simulink model "Simulacao"  (Simulink 8.2)
settings: Solver=ode4  SolverMode=SingleTasking  StartTime=0.0  StopTime=20  FixedStep=0.01  RelTol=1e-3
InitFcn:
  | Main
values from neighbouring files (symbols this model uses):
  T = 1    [Main.m]
  xk0 = [3; 5]    [Main.m]
undefined symbols (not defined in the file or in its folder): A1, B1, C, D
undefined symbols (not defined in the file): A, B, Umax
settings Model: Creator=Kawakami  LastModifiedBy=Eduardo
settings DataIOCC: LimitDataPoints=off  SaveOutput=off  SaveTime=off  TimeSaveName=t  SignalLoggingName=sigsOut
settings OptimizationCC: BooleanDataType=off
settings DebuggingCC: SaveWithParameterizedLinksMsg=none  SignalResolutionControl=TryResolveAllWithWarning  SolverPrmCheckMsg=none  MultiTaskDSMMsg=warning  MultiTaskCondExecSysMsg=none
settings HardwareCC: TargetUnknown=on
settings RTWCC: IncludeERTFirstTime=on

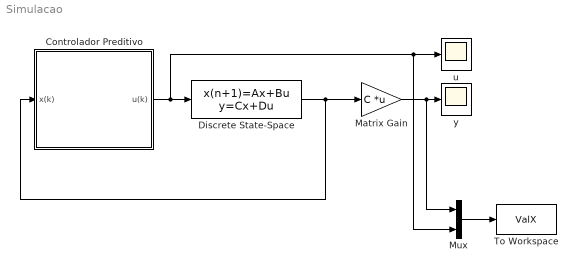
== system Simulacao ==
  "Controlador Preditivo  " : Subsystem  mask{A=A, B=B, Umax=Umax, T=T}
      mask prompts: A "Matriz Agregada A"; B "Matriz Agregada B"; Umax "Input Max"; T "T (passo da simulação)"
  Discrete State-Space : DiscreteStateSpace  A=A1  B=B1  C=C  D=D  X0=xk0
  Matrix Gain : Gain  Gain=C  Multiplication=Matrix(K*u)  SaturateOnIntegerOverflow=on  OutDataTypeStr=Inherit: Same as input  ParamDataTypeStr=Inherit: Same as input
  Mux : Mux  Inputs=2
  To Workspace : ToWorkspace  VariableName=ValX  SampleTime=-1  SaveFormat=Timeseries
  u : Scope
      settings: TimeRange=10  YMin=0.065  YMax=0.1075
  y : Scope
      settings: TimeRange=100  YMin=-191.5000000000001  YMax=48.49999999999989  SaveName=ScopeData2
  wires:
  "Controlador Preditivo  "/1(u(k)) -> Discrete State-Space/1, Mux/2, u/1
  Discrete State-Space/1 -> Matrix Gain/1, "Controlador Preditivo  "/1(x(k))
  Matrix Gain/1 -> Mux/1, y/1
  Mux/1 -> To Workspace/1

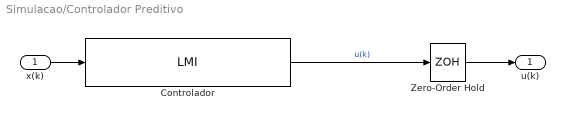
== system Simulacao/Controlador Preditivo   ==
  x(k) : Inport
  Controlador : S-Function  FunctionName=LMI  Parameters=A, B, Umax, T  EnableBusSupport=off
  Zero-Order Hold : ZeroOrderHold  SampleTime=T
  u(k) : Outport
  wires:
  Zero-Order Hold/1 -> u(k)/1
  Controlador/1 -> Zero-Order Hold/1  "u(k)"
  x(k)/1 -> Controlador/1
